simulink model "T4"  (R2025a)
settings: Solver=ode45  StartTime=0.0  StopTime=2  RelTol=1e-3  EnableMultiTasking=on
undefined symbols (not defined in the file): A, alpha, B, C, D, Kr, L, r, X0, x0
settings Model: Creator=andre.bergmann  LastModifiedBy=gmspe
settings SolverCC: AlgebraicLoopSolver=TrustRegion
settings DataIOCC: LimitDataPoints=on  SaveFormat=Array  ReturnWorkspaceOutputs=off
settings OptimizationCC: ExpressionDepthLimit=2147483647.0  LifeSpan=inf
settings DebuggingCC: UnderspecifiedInitializationDetection=Classic  MergeDetectMultiDrivingBlocksExec=none  SolverPrmCheckMsg=warning  UnconnectedInputMsg=warning  UnconnectedOutputMsg=warning  UnconnectedLineMsg=warning  StateNameClashWarn=warning  SFUnexpectedBacktrackingDiag=warning  SFNoUnconditionalDefaultTransitionDiag=warning  SFExecutionAtInitializationDiag=none  ArithmeticOperatorsInVariantConditions=warning
settings HardwareCC: ProdBitPerPointer=32.0  ProdBitPerSizeT=32.0  ProdBitPerPtrDiffT=32.0  ProdLargestAtomicFloat=None  ProdIntDivRoundTo=Undefined  ProdEndianess=Unspecified  ProdWordSize=32.0  ProdHWDeviceType=32-bit Generic
settings ModelReferenceCC: PropagateSignalLabelsOutOfModel=off
settings SFSimCC: SimUseLocalCustomCode=off  CustomCodeUndefinedFunction=UseInterfaceOnly
settings RTWCC: RTWUseLocalCustomCode=off  GPUComputeCapability=3.5
settings CodeAppCC: StateflowObjectComments=on
settings GRTTargetCC: TargetLangStandard=C89/C90 (ANSI)
settings ConfigComp: CovMetricSettings=dw  CovSaveCumulativeToWorkspaceVar=on  CovSaveSingleToWorkspaceVar=on  CovExternalEMLEnable=off

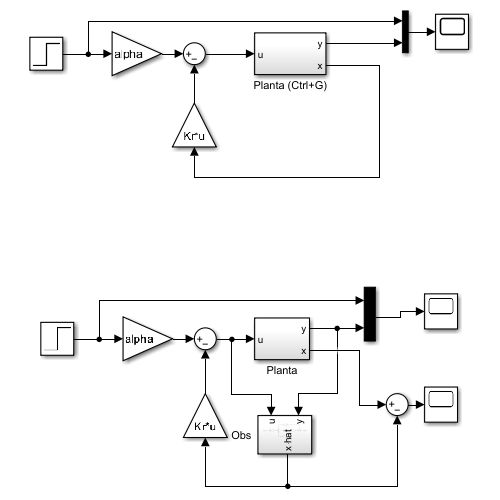
[thumbnail: Simulink's stored preview of the top-level diagram]
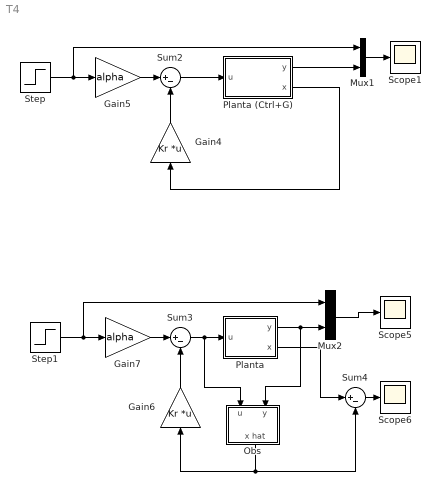
== system T4 ==
  Gain4 : Gain  Gain=Kr  Multiplication=Matrix(K*u)
  Gain5 : Gain  Gain=alpha
  Gain6 : Gain  Gain=Kr  Multiplication=Matrix(K*u)
  Gain7 : Gain  Gain=alpha
  Mux1 : Mux  Inputs=2
  Mux2 : Mux  Inputs=2
  Obs : Subsystem
  Planta : Subsystem
  Planta (Ctrl+G) : Subsystem
  Scope1 : Scope
      settings: ActiveDisplayYMinimum=-0.0012499999999999998  ActiveDisplayYMaximum=0.01125
  Scope5 : Scope
      settings: ActiveDisplayYMinimum=-0.001710313353439968  ActiveDisplayYMaximum=0.01149049024179721
  Scope6 : Scope
      settings: ActiveDisplayYMinimum=-1  ActiveDisplayYMaximum=1  DataLoggingVariableName=ScopeData2
  Step : Step  After=r  SampleTime=0
  Step1 : Step  After=r  SampleTime=0
  Sum2 : Sum  Inputs=|+-
  Sum3 : Sum  Inputs=|+-
  Sum4 : Sum  Inputs=|+-
  wires:
  Sum2/1 -> Planta (Ctrl+G)/1(u)
  Planta (Ctrl+G)/1(y) -> Mux1/2
  Planta (Ctrl+G)/2(x) -> Gain4/1
  Mux1/1 -> Scope1/1
  Gain4/1 -> Sum2/2
  Step/1 -> Mux1/1, Gain5/1
  Gain5/1 -> Sum2/1
  Step1/1 -> Mux2/1, Gain7/1
  Gain7/1 -> Sum3/1
  Mux2/1 -> Scope5/1
  Gain6/1 -> Sum3/2
  Sum3/1 -> Planta/1(u), Obs/1(u)
  Planta/1(y) -> Obs/2(y), Mux2/2
  Obs/1(x hat) -> Sum4/2, Gain6/1
  Planta/2(x) -> Sum4/1
  Sum4/1 -> Scope6/1

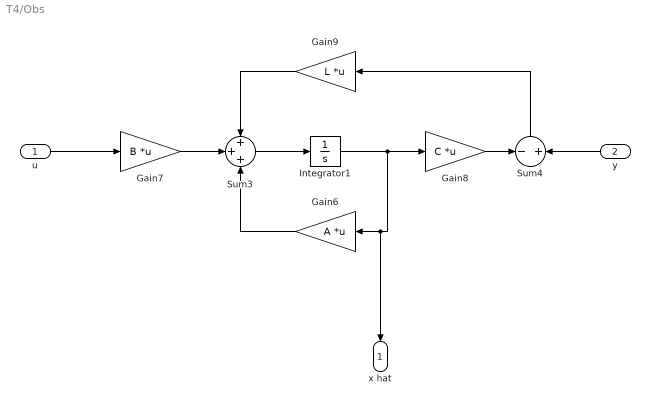
== system T4/Obs ==
  u : Inport
  y : Inport  Port=2
  Gain6 : Gain  Gain=A  Multiplication=Matrix(K*u)
  Gain7 : Gain  Gain=B  Multiplication=Matrix(K*u)
  Gain8 : Gain  Gain=C  Multiplication=Matrix(K*u)
  Gain9 : Gain  Gain=L  Multiplication=Matrix(K*u)
  Integrator1 : Integrator  InitialCondition=X0
  Sum3 : Sum  Inputs=+++
  Sum4 : Sum  Inputs=-|+
  x hat : Outport
  wires:
  Gain6/1 -> Sum3/3
  y/1 -> Sum4/2
  Integrator1/1 -> Gain6/1, x hat/1, Gain8/1
  Gain9/1 -> Sum3/1
  Sum3/1 -> Integrator1/1
  Gain7/1 -> Sum3/2
  Gain8/1 -> Sum4/1
  Sum4/1 -> Gain9/1
  u/1 -> Gain7/1

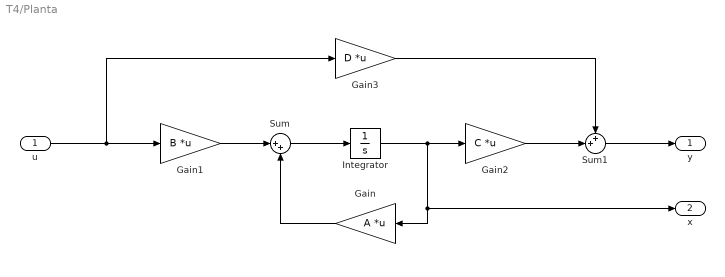
== system T4/Planta ==
  u : Inport
  Gain : Gain  Gain=A  Multiplication=Matrix(K*u)
  Gain1 : Gain  Gain=B  Multiplication=Matrix(K*u)
  Gain2 : Gain  Gain=C  Multiplication=Matrix(K*u)
  Gain3 : Gain  Gain=D  Multiplication=Matrix(K*u)
  Integrator : Integrator  InitialCondition=x0
  Sum : Sum  Inputs=|++
  Sum1 : Sum  Inputs=++|
  y : Outport
  x : Outport  Port=2
  wires:
  Gain1/1 -> Sum/1
  Gain2/1 -> Sum1/2
  u/1 -> Gain3/1, Gain1/1
  Sum1/1 -> y/1
  Sum/1 -> Integrator/1
  Gain3/1 -> Sum1/1
  Gain/1 -> Sum/2
  Integrator/1 -> x/1, Gain/1, Gain2/1

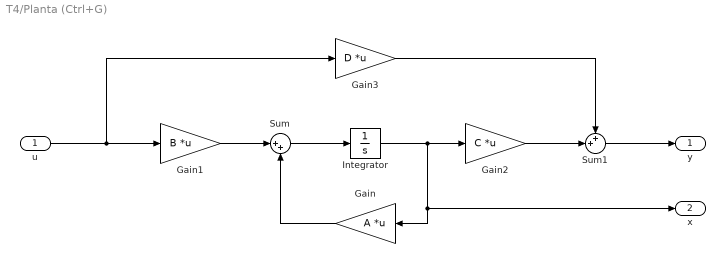
== system T4/Planta (Ctrl+G) ==
  u : Inport
  Gain : Gain  Gain=A  Multiplication=Matrix(K*u)
  Gain1 : Gain  Gain=B  Multiplication=Matrix(K*u)
  Gain2 : Gain  Gain=C  Multiplication=Matrix(K*u)
  Gain3 : Gain  Gain=D  Multiplication=Matrix(K*u)
  Integrator : Integrator  InitialCondition=x0
  Sum : Sum  Inputs=|++
  Sum1 : Sum  Inputs=++|
  y : Outport
  x : Outport  Port=2
  wires:
  Gain1/1 -> Sum/1
  Gain2/1 -> Sum1/2
  u/1 -> Gain3/1, Gain1/1
  Sum1/1 -> y/1
  Sum/1 -> Integrator/1
  Gain3/1 -> Sum1/1
  Gain/1 -> Sum/2
  Integrator/1 -> x/1, Gain/1, Gain2/1
